simulink model "gm_ImageProcessingNoShift_interface"  (R2023a)
settings: Solver=FixedStepDiscrete  StartTime=0.0  StopTime=2  RelTol=1e-3  EnableMultiTasking=on
undefined symbols (not defined in the file): gray
libraries: visionhdlio x6, hdlsllib x4, visionsources x4
Description:
  | Sobel Edge Detection Using the MATLAB(R) Function Block
  | This example shows how to use HDL Coder(TM) to check,
  | generate, and verify HDL code for a Sobel Edge Detection
  | block built using the MATLAB Function block.
settings Model: Creator=The MathWorks, Inc.  LastModifiedBy=ptl7263
settings SolverCC: AlgebraicLoopSolver=TrustRegion  PositivePriorityOrder=on
settings DataIOCC: LimitDataPoints=on  SaveFormat=Array  SignalLogging=off  ReturnWorkspaceOutputs=off
settings OptimizationCC: BlockReduction=off  ConditionallyExecuteInputs=off  EnhancedBackFolding=on  PassReuseOutputArgsAs=Individual arguments  ExpressionDepthLimit=2147483647  ZeroExternalMemoryAtStartup=off  ZeroInternalMemoryAtStartup=off  InitFltsAndDblsToZero=on  EfficientMapNaN2IntZero=off  MaxStackSize=64  OptimizeBlockOrder=speed  DifferentSizesBufferReuse=on  OptimizationCustomize=off  EfficientTunableParamExpr=on
settings DebuggingCC: AlgebraicLoopMsg=error  SaveWithParameterizedLinksMsg=none  UnderspecifiedInitializationDetection=Classic  MergeDetectMultiDrivingBlocksExec=none  SignalResolutionControl=TryResolveAllWithWarning  SingleTaskRateTransMsg=error  IntegerOverflowMsg=none  ParameterPrecisionLossMsg=none  ParameterTunabilityLossMsg=error  FcnCallInpInsideContextMsg=warning  UnconnectedInputMsg=warning  UnconnectedOutputMsg=warning  UnconnectedLineMsg=warning  AllowSymbolicDim=off  StateNameClashWarn=warning  StrictBusMsg=ErrorOnBusTreatedAsVector  SFUnexpectedBacktrackingDiag=warning  SFNoUnconditionalDefaultTransitionDiag=warning  SFExecutionAtInitializationDiag=none  IntegerSaturationMsg=none  ArithmeticOperatorsInVariantConditions=warning
settings HardwareCC: ProdBitPerPointer=32  ProdBitPerSizeT=32  ProdBitPerPtrDiffT=32  ProdLargestAtomicInteger=Long  ProdLargestAtomicFloat=Double  ProdWordSize=32  ProdLongLongMode=on  ProdHWDeviceType=ARM Compatible->ARM Cortex  TargetHWDeviceType=32-bit Generic
settings ModelReferenceCC: EnableRefExpFcnMdlSchedulingChecks=on  ModelReferenceNumInstancesAllowed=Single  PropagateSignalLabelsOutOfModel=off
settings SFSimCC: SimUseLocalCustomCode=off  MATLABDynamicMemAlloc=off  CustomCodeUndefinedFunction=UseInterfaceOnly
settings RTWCC: Description=Embedded Coder  SystemTargetFile=ert.tlc  HardwareBoard=Xilinx Zynq-7000 based board  TLCOptions="-aInlineSetEventsForThisBaseRateFcn=TLC_FALSE -aSuppressMultiTaskScheduler=TLC_FALSE  -aRateBasedStepFcn=0"  TemplateMakefile=ert_default_tmf  RTWUseLocalCustomCode=off  Toolchain=Linaro AArch32 Linux v6.3.1  DLArmComputeVersion=19.05
settings CodeAppCC: ForceParamTrailComments=on  IgnoreCustomStorageClasses=off  OperatorAnnotations=on  SimulinkDataObjDesc=on  SFDataObjDesc=on  InsertBlockDesc=on
settings ConfigComp: CovMetricSettings=dw  CovSaveCumulativeToWorkspaceVar=on  CovSaveSingleToWorkspaceVar=on  CovExternalEMLEnable=off

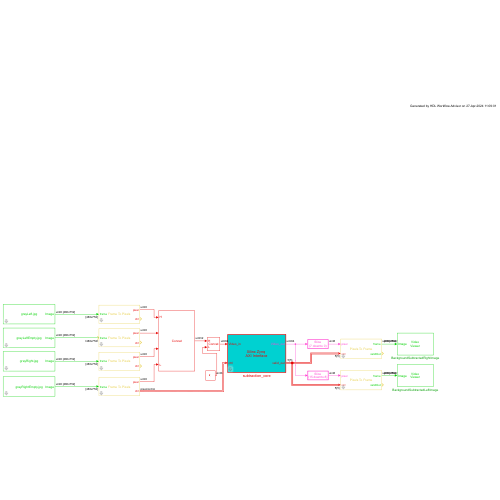
[thumbnail: Simulink's stored preview of the top-level diagram]
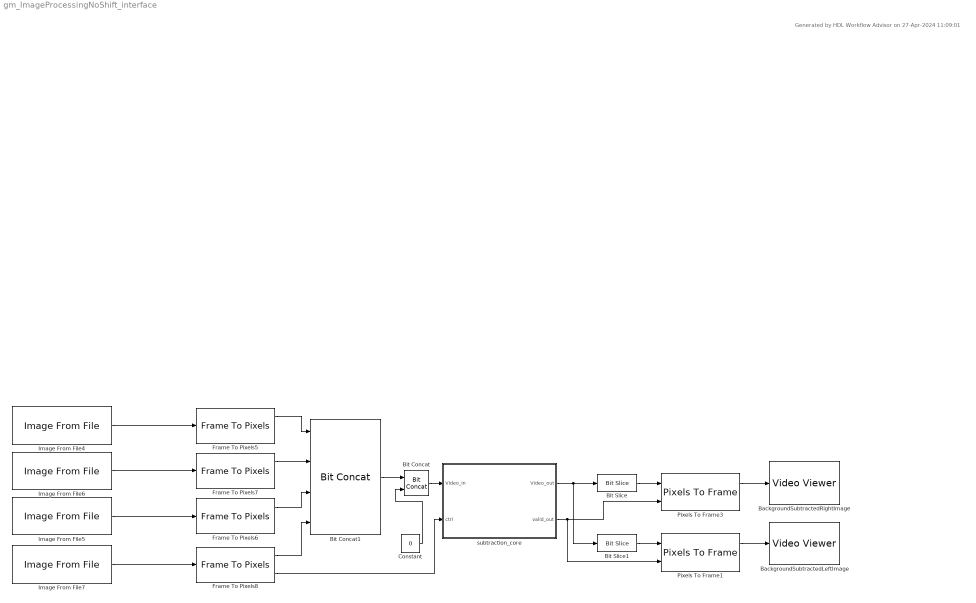
== system gm_ImageProcessingNoShift_interface ==
  note: Generated by HDL Workflow Advisor on 27-Apr-2024 11:09:01
  BackgroundSubtractedLeftImage : VideoViewer  colormapValue=gray(256)  FigPos=[1 1078 913 388]
  BackgroundSubtractedRightImage : VideoViewer  colormapValue=gray(256)  FigPos=[1 1078 913 388]
  Bit Concat : hdlsllib/Logic and Bit Operations/Bit Concat  numInputs=2
  Bit Concat1 : hdlsllib/Logic and Bit Operations/Bit Concat  numInputs=4
  Bit Slice : hdlsllib/Logic and Bit Operations/Bit Slice  lidx=7  ridx=0
  Bit Slice1 : hdlsllib/Logic and Bit Operations/Bit Slice  lidx=15  ridx=8
  Constant : Constant  Value=0  OutDataTypeStr=uint32  SampleTime=-1
  Frame To Pixels{5..8} (4 alike) : visionhdlio/Frame To Pixels  NumComponents=1  NumPixels=1  VideoFormat=Custom  ActivePixelsPerLine=R  ActiveVideoLines=C  TotalPixelsPerLine=R  TotalVideoLines=C  StartingActiveLine=1  FrontPorch=0  SampleTime=0  VideoFormatCache=Custom  ActivePixelsPerLineCache=R  ActiveVideoLinesCache=C  TotalPixelsPerLineCache=R  TotalVideoLinesCache=C  StartingActiveLineCache=1  FrontPorchCache=0
  Image From File4 : visionsources/Image From File  Tag=vipblks_nd  FileName=grayLeft.jpg  Ts=1  imagePorts=One multidimensional signal  OutPortLabels=R|G|B  ImageDataType=Inherit from input image  sdImageDataType=uint(8)  Signed=on  WordLength=16  FractionLengthMode=User-defined  FractionLength=15
  Image From File5 : visionsources/Image From File  Tag=vipblks_nd  FileName=grayRight.jpg  Ts=1  imagePorts=One multidimensional signal  OutPortLabels=R|G|B  ImageDataType=Inherit from input image  sdImageDataType=uint(8)  Signed=on  WordLength=16  FractionLengthMode=User-defined  FractionLength=15
  Image From File6 : visionsources/Image From File  Tag=vipblks_nd  FileName=grayLeftEmpty.jpg  Ts=1  imagePorts=One multidimensional signal  OutPortLabels=R|G|B  ImageDataType=Inherit from input image  sdImageDataType=uint(8)  Signed=on  WordLength=16  FractionLengthMode=User-defined  FractionLength=15
  Image From File7 : visionsources/Image From File  Tag=vipblks_nd  FileName=grayRightEmpty.jpg  Ts=1  imagePorts=One multidimensional signal  OutPortLabels=R|G|B  ImageDataType=Inherit from input image  sdImageDataType=uint(8)  Signed=on  WordLength=16  FractionLengthMode=User-defined  FractionLength=15
  Pixels To Frame1 : visionhdlio/Pixels To Frame  NumComponents=1  NumPixels=1  VideoFormat=Custom  ActivePixelsPerLine=R  ActiveVideoLines=C  TotalPixelsPerLine=R  TotalVideoLines=C  VideoFormatCache=Custom  ActivePixelsPerLineCache=R  ActiveVideoLinesCache=C  TotalPixelsPerLineCache=R  TotalVideoLinesCache=C
  Pixels To Frame3 : visionhdlio/Pixels To Frame  NumComponents=1  NumPixels=1  VideoFormat=Custom  ActivePixelsPerLine=R  ActiveVideoLines=C  TotalPixelsPerLine=R  TotalVideoLines=C  VideoFormatCache=Custom  ActivePixelsPerLineCache=R  ActiveVideoLinesCache=C  TotalPixelsPerLineCache=R  TotalVideoLinesCache=C
  subtraction_core : Subsystem  TreatAsAtomicUnit=on  mask(AXI4-Lite/AXI4 Interface){}
      mask help:
      | This is an automatically generated subsystem block.
      | This contains the AXI interface blocks that communicate with the subtracti_ip IPCore generated from ImageProcessingNoShift/subtraction_core subsystem.
      mask Display: disp(sprintf('Xilinx Zynq \nAXI Interface'));
  wires:
  Pixels To Frame1/1 -> BackgroundSubtractedLeftImage/1
  Pixels To Frame3/1 -> BackgroundSubtractedRightImage/1
  Bit Slice1/1 -> Pixels To Frame1/1
  Bit Slice/1 -> Pixels To Frame3/1
  subtraction_core/1(Video_out) -> Bit Slice1/1, Bit Slice/1
  subtraction_core/2(valid_out) -> Pixels To Frame1/2, Pixels To Frame3/2
  Bit Concat/1 -> subtraction_core/1(Video_in)
  Bit Concat1/1 -> Bit Concat/1
  Frame To Pixels8/2 -> subtraction_core/2(ctrl)
  Frame To Pixels8/1 -> Bit Concat1/4
  Frame To Pixels6/1 -> Bit Concat1/3
  Image From File7/1 -> Frame To Pixels8/1
  Image From File5/1 -> Frame To Pixels6/1
  Image From File6/1 -> Frame To Pixels7/1
  Image From File4/1 -> Frame To Pixels5/1
  Frame To Pixels5/1 -> Bit Concat1/1
  Frame To Pixels7/1 -> Bit Concat1/2
  Constant/1 -> Bit Concat/2

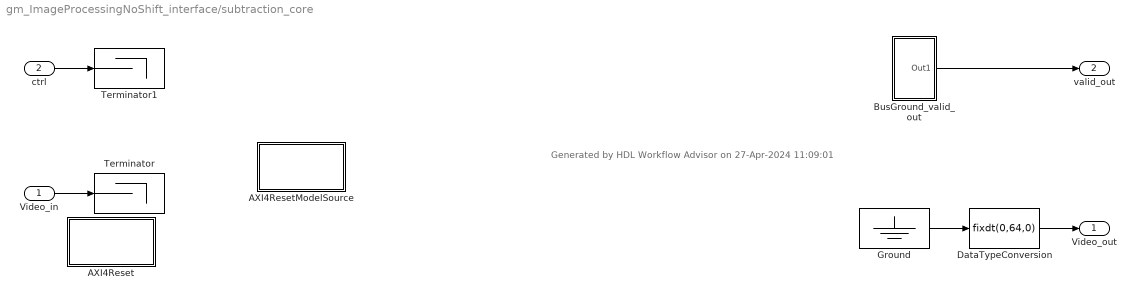
== system gm_ImageProcessingNoShift_interface/subtraction_core ==
  note: Generated by HDL Workflow Advisor on 27-Apr-2024 11:09:01
  Video_in : Inport
  ctrl : Inport  Port=2
  AXI4Reset : Subsystem  mask(System Start){ShowInLibBrowser=0}
      mask prompts: ShowInLibBrowser "Simulink:masks:CustCodeMaskParam1_MP"
      settings: CopyFcn=cccopyfcn(gcb)  OpenFcn=ccopenfcn('System Start Function')
      mask Help: eval('feval(''rtwprivate'',''rtwhelpview'',''rtw_sys_start_block'')');
      mask Display: disp('System\nStart');
  AXI4ResetModelSource : Subsystem  mask(Model Source){ShowInLibBrowser=0}
      mask prompts: ShowInLibBrowser "Simulink:masks:CustCodeMaskParam1_MP"
      settings: CopyFcn=cccopyfcn(gcb)  OpenFcn=ccopenfcn('Model Source')
      mask Help: eval('feval(''rtwprivate'',''rtwhelpview'',''rtw_model_source_block'')');
      mask Display: disp('Model\nSource');
  BusGround_valid_out : Subsystem
  DataTypeConversion : DataTypeConversion  OutDataTypeStr=fixdt(0,64,0)  ConvertRealWorld=Stored Integer (SI)  SaturateOnIntegerOverflow=off  RndMeth=Floor
  Ground : Ground
  Terminator : Terminator
  Terminator1 : Terminator
  Video_out : Outport  VectorParamsAs1DForOutWhenUnconnected=off
  valid_out : Outport  Port=2  VectorParamsAs1DForOutWhenUnconnected=off
  wires:
  Video_in/1 -> Terminator/1
  ctrl/1 -> Terminator1/1
  DataTypeConversion/1 -> Video_out/1
  Ground/1 -> DataTypeConversion/1
  BusGround_valid_out/1(Out1) -> valid_out/1

== system gm_ImageProcessingNoShift_interface/subtraction_core/AXI4Reset ==

== system gm_ImageProcessingNoShift_interface/subtraction_core/AXI4ResetModelSource ==

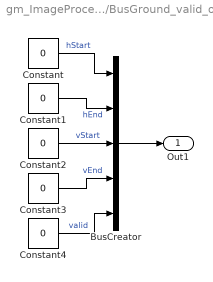
== system gm_ImageProcessingNoShift_interface/subtraction_core/BusGround_valid_out ==
  BusCreator : BusCreator  Inputs=5
  Constant{,1..4} (5 alike) : Constant  Value=0  OutDataTypeStr=fixdt('boolean')  SampleTime=-1
  Out1 : Outport
  wires:
  Constant2/1 -> BusCreator/3  "vStart"
  Constant/1 -> BusCreator/1  "hStart"
  Constant4/1 -> BusCreator/5  "valid"
  Constant3/1 -> BusCreator/4  "vEnd"
  Constant1/1 -> BusCreator/2  "hEnd"
  BusCreator/1 -> Out1/1
